simulink model "controller_tuning"  (R2020a)
settings: Solver=VariableStepAuto  StartTime=0.0  StopTime=10.0  RelTol=1e-3
model workspace (MAT data in the model file):
  DM0 = [1.094  0.6666; 0.3097  0.2601; -0.2633  0.1218; -0.351  0.6966; -0.105  0.4764; -0.3242  -0.09756; 0.796  1.029; 0.2022  0.05678]
  G = tf
  G.Variable_ = 'z^-1'
  G.InputName_ = ["TRIlong"; "TRIlat"; "TRImed"; "BIClong"; "BICshort"; "BRA"; "shoulder reserve"; "elbow reserve"]
  G.InputUnit_ = [""; ""; ""; ""; ""; ""; ""; ""]
  G.OutputName_ = ["y(1)"; "y(2)"]
  G.OutputUnit_ = [""; ""]
  G.Name_ = 'sys9'
  G.IOSize_ = [2 8]
  G.Data_ = ltipack.tfdata
  G.Data_.num{1,1} = [0 -0.00125852005922 -0.00123969277085 0.00578303193573 -0.00214602833438 -0.00815494705012 0.0108004774488 -0.0048408303984 0.000317114183203 0.000131024551851]
  G.Data_.num{2,1} = [0 -1.78877461201 3.42269225285 -0.172240731746 -4.80550166472 5.61225680994 -4.36357973513 4.54900861654 -3.65235478567 1.19849686118]
  G.Data_.num{1,2} = [0 0.0298263266299 -0.05603494088 0.00949204168653 0.0313146678964 0.0133073865004 -0.0557080006374 0.0253256021985 0.0130251372604 -0.00928844893676]
  G.Data_.num{2,2} = [0 6.78283210007 -16.0998067341 6.29571390083 14.1517930939 -18.338769316 15.0577755183 -18.5075343986 16.3599337451 -5.7019804007]
  G.Data_.num{1,3} = [0 -0.0274580753918 0.046649778889 0.000219075801083 -0.0277627580393 -0.0275977505479 0.0648552045639 -0.0245133704063 -0.0166522040766 0.0113266772791]
  G.Data_.num{2,3} = [0 -7.30509401763 17.0847598655 -6.42957231831 -15.715976147 21.2307859184 -18.337456702 20.0855611081 -15.011225285 4.39826116622]
  G.Data_.num{1,4} = [0 -0.000892023297362 0.00174771311212 -5.02626521608e-05 -0.0020036315742 0.000859099403795 0.00133312807044 -0.00136865103822 0.000340032171244 3.78324308943e-06]
  G.Data_.num{2,4} = [0 -0.125954978135 0.32847363204 -0.172297865784 -0.275766220436 0.382500727314 -0.353411491272 0.691035305427 -0.761724888908 0.287146907417]
  G.Data_.num{1,5} = [0 -0.00769047181105 0.0200271669402 -0.0171499217797 -0.0017607521966 0.0110210193173 -0.00610528432784 0.00273344797859 -0.00365422344999 0.00163564285109]
  G.Data_.num{2,5} = [0 -0.595361713331 0.656194025324 -0.708001157476 2.48746014578 -4.19785050587 4.1108803772 -2.57579141198 0.647172525737 0.175305987775]
  G.Data_.num{1,6} = [0 0.0106958101176 -0.0156960010931 -0.00894123836845 0.0450636393289 -0.0437527767735 0.00495298305972 0.0244991267401 -0.0226105055791 0.00832888442118]
  G.Data_.num{2,6} = [0 7.63813053731 -16.0040222918 8.78360619231 -0.807775906777 6.14010716966 -5.6743918868 -9.51802269738 16.2988522235 -6.85648806661]
  G.Data_.num{1,7} = [0 0.0096689266463 -0.0352403034351 0.0530644872076 -0.0277649986769 -0.0217759796863 0.0428504114816 -0.0292889462176 0.0114475784774 -0.00257741725747]
  G.Data_.num{2,7} = [0 0.705264065553 0.136559901801 -0.466566874265 -6.64333058905 16.0560931678 -19.450434008 16.8727296984 -9.81674981039 2.60643162571]
  G.Data_.num{1,8} = [0 -0.288241005177 0.902709439389 -0.75873047364 -0.65955283102 1.79703167037 -1.30558234166 0.128044890915 0.32409931535 -0.138466743751]
  G.Data_.num{2,8} = [0 -43.8066730621 155.493123951 -278.509814702 470.342011324 -720.208447619 693.978256442 -309.311208705 0.183476450966 31.8392957397]
  G.Data_.den{1,1} = [1 -3.44110275617 4.07951037305 -1.37498385443 -0.519157706389 -0.282617710591 0.517166185053 0.784556988423 -1.17222288306 0.408852682884]
  G.Data_.den{2,1} = [1 -3.44110275617 4.07951037305 -1.37498385443 -0.519157706389 -0.282617710591 0.517166185053 0.784556988423 -1.17222288306 0.408852682884]
  G.Data_.den{1,2} = [1 -3.44110275617 4.07951037305 -1.37498385443 -0.519157706389 -0.282617710591 0.517166185053 0.784556988423 -1.17222288306 0.408852682884]
  G.Data_.den{2,2} = [1 -3.44110275617 4.07951037305 -1.37498385443 -0.519157706389 -0.282617710591 0.517166185053 0.784556988423 -1.17222288306 0.408852682884]
  G.Data_.den{1,3} = [1 -3.44110275617 4.07951037305 -1.37498385443 -0.519157706389 -0.282617710591 0.517166185053 0.784556988423 -1.17222288306 0.408852682884]
  G.Data_.den{2,3} = [1 -3.44110275617 4.07951037305 -1.37498385443 -0.519157706389 -0.282617710591 0.517166185053 0.784556988423 -1.17222288306 0.408852682884]
  G.Data_.den{1,4} = [1 -3.44110275617 4.07951037305 -1.37498385443 -0.519157706389 -0.282617710591 0.517166185053 0.784556988423 -1.17222288306 0.408852682884]
  G.Data_.den{2,4} = [1 -3.44110275617 4.07951037305 -1.37498385443 -0.519157706389 -0.282617710591 0.517166185053 0.784556988423 -1.17222288306 0.408852682884]
  G.Data_.den{1,5} = [1 -3.44110275617 4.07951037305 -1.37498385443 -0.519157706389 -0.282617710591 0.517166185053 0.784556988423 -1.17222288306 0.408852682884]
  G.Data_.den{2,5} = [1 -3.44110275617 4.07951037305 -1.37498385443 -0.519157706389 -0.282617710591 0.517166185053 0.784556988423 -1.17222288306 0.408852682884]
  G.Data_.den{1,6} = [1 -3.44110275617 4.07951037305 -1.37498385443 -0.519157706389 -0.282617710591 0.517166185053 0.784556988423 -1.17222288306 0.408852682884]
  G.Data_.den{2,6} = [1 -3.44110275617 4.07951037305 -1.37498385443 -0.519157706389 -0.282617710591 0.517166185053 0.784556988423 -1.17222288306 0.408852682884]
  G.Data_.den{1,7} = [1 -3.44110275617 4.07951037305 -1.37498385443 -0.519157706389 -0.282617710591 0.517166185053 0.784556988423 -1.17222288306 0.408852682884]
  G.Data_.den{2,7} = [1 -3.44110275617 4.07951037305 -1.37498385443 -0.519157706389 -0.282617710591 0.517166185053 0.784556988423 -1.17222288306 0.408852682884]
  G.Data_.den{1,8} = [1 -3.44110275617 4.07951037305 -1.37498385443 -0.519157706389 -0.282617710591 0.517166185053 0.784556988423 -1.17222288306 0.408852682884]
  G.Data_.den{2,8} = [1 -3.44110275617 4.07951037305 -1.37498385443 -0.519157706389 -0.282617710591 0.517166185053 0.784556988423 -1.17222288306 0.408852682884]
  G.Data_.Delay.Input = [0; 0; 0; 0; 0; 0; 0; 0]
  G.Data_.Delay.Output = [0; 0]
  G.Data_.Delay.IO = [0  0  0  0  0  0  0  0; 0  0  0  0  0  0  0  0]
  G.Data_.Ts = 0.001
  Ts = 0.001
  controllers{1} = tunablePID
  controllers{1}.Kp_ = param.Continuous
  controllers{1}.Kp_.Size_ = [1 1]
  controllers{1}.Kp_.Value_ = 0
  controllers{1}.Kp_.pID = paramid.Variable
  controllers{1}.Kp_.pID.Name = 'Kp'
  controllers{1}.Ki_ = param.Continuous
  controllers{1}.Ki_.Size_ = [1 1]
  controllers{1}.Ki_.Value_ = 0.001
  controllers{1}.Ki_.pID = paramid.Variable
  controllers{1}.Ki_.pID.Name = 'Ki'
  controllers{1}.Kd_ = param.Continuous
  controllers{1}.Kd_.Free_ = 0
  controllers{1}.Kd_.Size_ = [1 1]
  controllers{1}.Kd_.Value_ = 0
  controllers{1}.Kd_.pID = paramid.Variable
  controllers{1}.Kd_.pID.Name = 'Kd'
  controllers{1}.Tf_ = param.Continuous
  controllers{1}.Tf_.Minimum_ = 0
  controllers{1}.Tf_.Free_ = 0
  controllers{1}.Tf_.Size_ = [1 1]
  controllers{1}.Tf_.Value_ = 1
  controllers{1}.Tf_.pID = paramid.Variable
  controllers{1}.Tf_.pID.Name = 'Tf'
  controllers{1}.Name_ = 'PI1'
  controllers{1}.IOSize_ = [1 1]
  controllers{1}.Ts_ = 0.001
  controllers{1}.InputName_ = "p(1)"
  controllers{1}.OutputName_ = "TRIlong"
  controllers{2} = tunablePID
  controllers{2}.Kp_ = param.Continuous
  controllers{2}.Kp_.Size_ = [1 1]
  controllers{2}.Kp_.Value_ = 0
  controllers{2}.Kp_.pID = paramid.Variable
  controllers{2}.Kp_.pID.Name = 'Kp'
  controllers{2}.Ki_ = param.Continuous
  controllers{2}.Ki_.Size_ = [1 1]
  controllers{2}.Ki_.Value_ = 0.001
  controllers{2}.Ki_.pID = paramid.Variable
  controllers{2}.Ki_.pID.Name = 'Ki'
  controllers{2}.Kd_ = param.Continuous
  controllers{2}.Kd_.Free_ = 0
  controllers{2}.Kd_.Size_ = [1 1]
  controllers{2}.Kd_.Value_ = 0
  controllers{2}.Kd_.pID = paramid.Variable
  controllers{2}.Kd_.pID.Name = 'Kd'
  controllers{2}.Tf_ = param.Continuous
  controllers{2}.Tf_.Minimum_ = 0
  controllers{2}.Tf_.Free_ = 0
  controllers{2}.Tf_.Size_ = [1 1]
  controllers{2}.Tf_.Value_ = 1
  controllers{2}.Tf_.pID = paramid.Variable
  controllers{2}.Tf_.pID.Name = 'Tf'
  controllers{2}.Name_ = 'PI2'
  controllers{2}.IOSize_ = [1 1]
  controllers{2}.Ts_ = 0.001
  controllers{2}.InputName_ = "p(2)"
  controllers{2}.OutputName_ = "TRIlat"
  controllers{3} = tunablePID
  controllers{3}.Kp_ = param.Continuous
  controllers{3}.Kp_.Size_ = [1 1]
  controllers{3}.Kp_.Value_ = 0
  controllers{3}.Kp_.pID = paramid.Variable
  controllers{3}.Kp_.pID.Name = 'Kp'
  controllers{3}.Ki_ = param.Continuous
  controllers{3}.Ki_.Size_ = [1 1]
  controllers{3}.Ki_.Value_ = 0.001
  controllers{3}.Ki_.pID = paramid.Variable
  controllers{3}.Ki_.pID.Name = 'Ki'
  controllers{3}.Kd_ = param.Continuous
  controllers{3}.Kd_.Free_ = 0
  controllers{3}.Kd_.Size_ = [1 1]
  controllers{3}.Kd_.Value_ = 0
  controllers{3}.Kd_.pID = paramid.Variable
  controllers{3}.Kd_.pID.Name = 'Kd'
  controllers{3}.Tf_ = param.Continuous
  controllers{3}.Tf_.Minimum_ = 0
  controllers{3}.Tf_.Free_ = 0
  controllers{3}.Tf_.Size_ = [1 1]
  controllers{3}.Tf_.Value_ = 1
  controllers{3}.Tf_.pID = paramid.Variable
  controllers{3}.Tf_.pID.Name = 'Tf'
  controllers{3}.Name_ = 'PI3'
  controllers{3}.IOSize_ = [1 1]
  controllers{3}.Ts_ = 0.001
  controllers{3}.InputName_ = "p(3)"
  controllers{3}.OutputName_ = "TRImed"
  controllers{4} = tunablePID
  controllers{4}.Kp_ = param.Continuous
  controllers{4}.Kp_.Size_ = [1 1]
  controllers{4}.Kp_.Value_ = 0
  controllers{4}.Kp_.pID = paramid.Variable
  controllers{4}.Kp_.pID.Name = 'Kp'
  controllers{4}.Ki_ = param.Continuous
  controllers{4}.Ki_.Size_ = [1 1]
  controllers{4}.Ki_.Value_ = 0.001
  controllers{4}.Ki_.pID = paramid.Variable
  controllers{4}.Ki_.pID.Name = 'Ki'
  controllers{4}.Kd_ = param.Continuous
  controllers{4}.Kd_.Free_ = 0
  controllers{4}.Kd_.Size_ = [1 1]
  controllers{4}.Kd_.Value_ = 0
  controllers{4}.Kd_.pID = paramid.Variable
  controllers{4}.Kd_.pID.Name = 'Kd'
  controllers{4}.Tf_ = param.Continuous
  controllers{4}.Tf_.Minimum_ = 0
  controllers{4}.Tf_.Free_ = 0
  controllers{4}.Tf_.Size_ = [1 1]
  controllers{4}.Tf_.Value_ = 1
  controllers{4}.Tf_.pID = paramid.Variable
  controllers{4}.Tf_.pID.Name = 'Tf'
  controllers{4}.Name_ = 'PI4'
  controllers{4}.IOSize_ = [1 1]
  controllers{4}.Ts_ = 0.001
  controllers{4}.InputName_ = "p(4)"
  controllers{4}.OutputName_ = "BIClong"
  controllers{5} = tunablePID
  controllers{5}.Kp_ = param.Continuous
  controllers{5}.Kp_.Size_ = [1 1]
  controllers{5}.Kp_.Value_ = 0
  controllers{5}.Kp_.pID = paramid.Variable
  controllers{5}.Kp_.pID.Name = 'Kp'
  controllers{5}.Ki_ = param.Continuous
  controllers{5}.Ki_.Size_ = [1 1]
  controllers{5}.Ki_.Value_ = 0.001
  controllers{5}.Ki_.pID = paramid.Variable
  controllers{5}.Ki_.pID.Name = 'Ki'
  controllers{5}.Kd_ = param.Continuous
  controllers{5}.Kd_.Free_ = 0
  controllers{5}.Kd_.Size_ = [1 1]
  controllers{5}.Kd_.Value_ = 0
  controllers{5}.Kd_.pID = paramid.Variable
  controllers{5}.Kd_.pID.Name = 'Kd'
  controllers{5}.Tf_ = param.Continuous
  controllers{5}.Tf_.Minimum_ = 0
  controllers{5}.Tf_.Free_ = 0
  controllers{5}.Tf_.Size_ = [1 1]
  controllers{5}.Tf_.Value_ = 1
  controllers{5}.Tf_.pID = paramid.Variable
  controllers{5}.Tf_.pID.Name = 'Tf'
  controllers{5}.Name_ = 'PI5'
  controllers{5}.IOSize_ = [1 1]
  controllers{5}.Ts_ = 0.001
  controllers{5}.InputName_ = "p(5)"
  controllers{5}.OutputName_ = "BICshort"
  controllers{6} = tunablePID
  controllers{6}.Kp_ = param.Continuous
  controllers{6}.Kp_.Size_ = [1 1]
  controllers{6}.Kp_.Value_ = 0
  controllers{6}.Kp_.pID = paramid.Variable
  controllers{6}.Kp_.pID.Name = 'Kp'
  controllers{6}.Ki_ = param.Continuous
  controllers{6}.Ki_.Size_ = [1 1]
  controllers{6}.Ki_.Value_ = 0.001
  controllers{6}.Ki_.pID = paramid.Variable
  controllers{6}.Ki_.pID.Name = 'Ki'
  controllers{6}.Kd_ = param.Continuous
  controllers{6}.Kd_.Free_ = 0
  controllers{6}.Kd_.Size_ = [1 1]
  controllers{6}.Kd_.Value_ = 0
  controllers{6}.Kd_.pID = paramid.Variable
  controllers{6}.Kd_.pID.Name = 'Kd'
  controllers{6}.Tf_ = param.Continuous
  controllers{6}.Tf_.Minimum_ = 0
  controllers{6}.Tf_.Free_ = 0
  controllers{6}.Tf_.Size_ = [1 1]
  controllers{6}.Tf_.Value_ = 1
  controllers{6}.Tf_.pID = paramid.Variable
  controllers{6}.Tf_.pID.Name = 'Tf'
  controllers{6}.Name_ = 'PI6'
  controllers{6}.IOSize_ = [1 1]
  controllers{6}.Ts_ = 0.001
  controllers{6}.InputName_ = "p(6)"
  controllers{6}.OutputName_ = "BRA"
  controllers{7} = tunablePID
  controllers{7}.Kp_ = param.Continuous
  controllers{7}.Kp_.Size_ = [1 1]
  controllers{7}.Kp_.Value_ = 0
  controllers{7}.Kp_.pID = paramid.Variable
  controllers{7}.Kp_.pID.Name = 'Kp'
  controllers{7}.Ki_ = param.Continuous
  controllers{7}.Ki_.Size_ = [1 1]
  controllers{7}.Ki_.Value_ = 0.001
  controllers{7}.Ki_.pID = paramid.Variable
  controllers{7}.Ki_.pID.Name = 'Ki'
  controllers{7}.Kd_ = param.Continuous
  controllers{7}.Kd_.Free_ = 0
  controllers{7}.Kd_.Size_ = [1 1]
  controllers{7}.Kd_.Value_ = 0
  controllers{7}.Kd_.pID = paramid.Variable
  controllers{7}.Kd_.pID.Name = 'Kd'
  controllers{7}.Tf_ = param.Continuous
  controllers{7}.Tf_.Minimum_ = 0
  controllers{7}.Tf_.Free_ = 0
  controllers{7}.Tf_.Size_ = [1 1]
  controllers{7}.Tf_.Value_ = 1
  controllers{7}.Tf_.pID = paramid.Variable
  controllers{7}.Tf_.pID.Name = 'Tf'
  controllers{7}.Name_ = 'PI7'
  controllers{7}.IOSize_ = [1 1]
  controllers{7}.Ts_ = 0.001
  controllers{7}.InputName_ = "p(7)"
  controllers{7}.OutputName_ = "shoulder reserve"
  controllers{8} = tunablePID
  controllers{8}.Kp_ = param.Continuous
  controllers{8}.Kp_.Size_ = [1 1]
  controllers{8}.Kp_.Value_ = 0
  controllers{8}.Kp_.pID = paramid.Variable
  controllers{8}.Kp_.pID.Name = 'Kp'
  controllers{8}.Ki_ = param.Continuous
  controllers{8}.Ki_.Size_ = [1 1]
  controllers{8}.Ki_.Value_ = 0.001
  controllers{8}.Ki_.pID = paramid.Variable
  controllers{8}.Ki_.pID.Name = 'Ki'
  controllers{8}.Kd_ = param.Continuous
  controllers{8}.Kd_.Free_ = 0
  controllers{8}.Kd_.Size_ = [1 1]
  controllers{8}.Kd_.Value_ = 0
  controllers{8}.Kd_.pID = paramid.Variable
  controllers{8}.Kd_.pID.Name = 'Kd'
  controllers{8}.Tf_ = param.Continuous
  controllers{8}.Tf_.Minimum_ = 0
  controllers{8}.Tf_.Free_ = 0
  controllers{8}.Tf_.Size_ = [1 1]
  controllers{8}.Tf_.Value_ = 1
  controllers{8}.Tf_.pID = paramid.Variable
  controllers{8}.Tf_.pID.Name = 'Tf'
  controllers{8}.Name_ = 'PI8'
  controllers{8}.IOSize_ = [1 1]
  controllers{8}.Ts_ = 0.001
  controllers{8}.InputName_ = "p(8)"
  controllers{8}.OutputName_ = "elbow reserve"
values from neighbouring files (symbols this model uses):
  D = tunableGain('Decoupler', numinputs, numoutputs)    [closed_loop_controller_tuning.m]    (also in steptester.m)
  G = sys_tf    [closed_loop_controller_tuning.m]    (also in steptester.m)
undefined symbols (not defined in the file or in its folder): Tdio
libraries: cstextras x20, simulink x16, simulink_extras x2
settings Model: Creator=Jaxton  LastModifiedBy=Jaxton

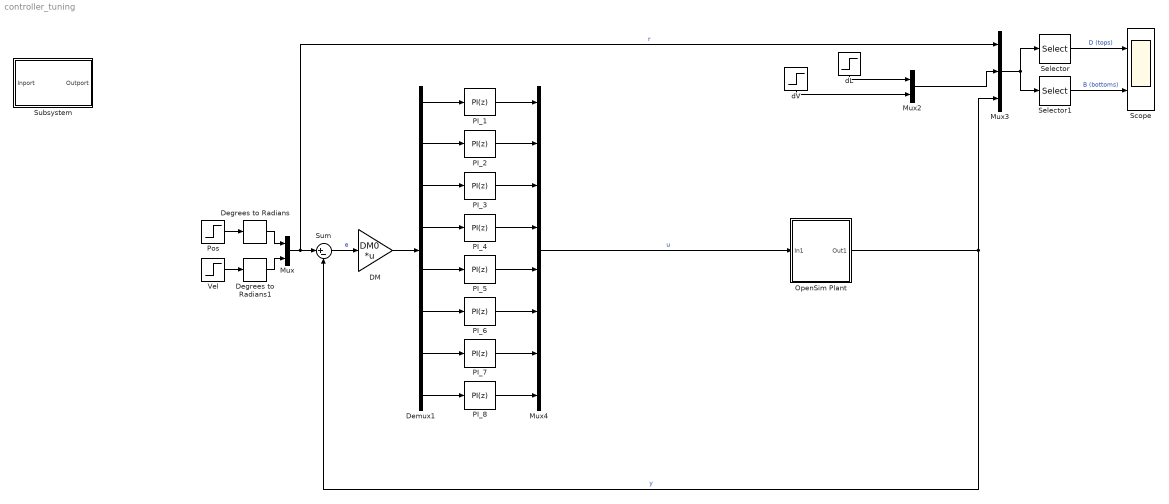
== system controller_tuning ==
  DM : Gain  Gain=DM0  Multiplication=Matrix(K*u)
  Degrees to Radians : simulink_extras/Transformations/Degrees to Radians
  Degrees to Radians1 : simulink_extras/Transformations/Degrees to Radians
  Demux1 : Demux  Outputs=8
  Mux : Mux  Inputs=2
  Mux2 : Mux  Inputs=2
  Mux3 : Mux  Inputs=3
  Mux4 : Mux  Inputs=8
  OpenSim Plant : Subsystem  BlockChoice=CSS  mask(LTI Block){sys=G, IC=[]}
      mask prompts: sys "Control:simulink:LTIMaskLabel1"; IC "Control:simulink:LTIMaskLabel2"
      mask help: Control:simulink:LTIMaskDescription
      mask init:
      | try
      |    % read data to initialize mask variables
      |    [D,Ts,Tdi,Tdo,Tdio,x0,sysname]=...
      |       ltimask('Initialize',gcb,sys,IC);
      |    % update contents
      |    model = bdroot;
      |    df = get_param(model,'dirty');
      |    ltimask('UpdateDiagram',gcb,D,Ts,Tdio);
      |    try      
      |       % Attempt to modify locked library -> error
      |       % Makes block show ??? when loading CSTBLOCKS
      |       % for the first time
      |       set_param(model,'dirty',df)
      |    end
      | catch ME
      |    sys = [];  IC = [];   sysname = '???';
      |    throw(ME)
      | end
      mask Help: eval('ctrlguihelp(''ltisystemblock'');')
      mask Callback sys: ltimask('MaskLTICallback',gcb);
      mask Display: disp(sysname)
  PI_1 : simulink/Continuous/PID Controller  Controller=PI  Form=Parallel  TimeDomain=Discrete-time  UseExternalTs=off  SampleTime=-1  IntegratorMethod=Forward Euler  FilterMethod=Forward Euler  ControllerParametersSource=internal  P=-0.385  I=-0.958  D=0  UseFilter=on  N=100  TunerSelectOption=Transfer Function Based (PID Tuner App)  InitialConditionSource=internal  InitialConditionForIntegrator=0  InitialConditionForFilter=0  DifferentiatorICPrevScaledInput=0  ExternalReset=none  TrackingMode=off  Kt=1  LimitOutput=off  UpperSaturationLimit=inf  LowerSaturationLimit=-inf  LinearizeAsGain=off  AntiWindupMode=none  Kb=1  POutMin=[]  POutMax=[]  IOutMin=[]  IOutMax=[]  DOutMin=[]  DOutMax=[]  NOutMin=[]  NOutMax=[]  SumOutMin=[]  SumOutMax=[]  SaturationOutMin=[]  SaturationOutMax=[]  PParamMin=[]  PParamMax=[]  IParamMin=[]  IParamMax=[]  DParamMin=[]  DParamMax=[]  NParamMin=[]  NParamMax=[]  KbParamMin=[]  KbParamMax=[]  KtParamMin=[]  KtParamMax=[]  KbOutMin=[]  KbOutMax=[]  KtOutMin=[]  KtOutMax=[]  IntegratorOutMin=[]  IntegratorOutMax=[]  FilterOutMin=[]  FilterOutMax=[]  SumI1OutMin=[]  SumI1OutMax=[]  SumI2OutMin=[]  SumI2OutMax=[]  SumI3OutMin=[]  SumI3OutMax=[]  SumI4OutMin=[]  SumI4OutMax=[]  SumDOutMin=[]  SumDOutMax=[]  DifferentiatorOutMin=[]  DifferentiatorOutMax=[]  FilterDiffOutCoefMin=[]  FilterDiffOutCoefMax=[]  ReciprocalOutMin=[]  ReciprocalOutMax=[]  SumDenOutMin=[]  SumDenOutMax=[]  SumNumOutMin=[]  SumNumOutMax=[]  DivideOutMin=[]  DivideOutMax=[]  UdiffTsProdOutMin=[]  UdiffTsProdOutMax=[]  NTsProdOutMin=[]  NTsProdOutMax=[]  UintegralTsProdOutMin=[]  UintegralTsProdOutMax=[]  UngainTsProdOutMin=[]  UngainTsProdOutMax=[]  IntegratorContinuousStateAttributes=''  IntegratorStateMustResolveToSignalObject=off  IntegratorRTWStateStorageClass=Auto  FilterContinuousStateAttributes=''  FilterStateMustResolveToSignalObject=off  FilterRTWStateStorageClass=Auto  ParallelPVariant=InternalParameters  IdealPVariant=Disabled  IVariant=InternalParameters  DVariant=Disabled  IntegratorVariant=Discrete  SatVariant=Disabled  AWVariant=Passthrough  PCopyVariant=Disabled  TRVariant=Disabled  FdbkBlocksVariant=Forward  IdealPFdbkVariant=Disabled  SatFdbkVariant=Disabled  DerivativeFilterVariant=Disabled  NVariant=Disabled  NCopyVariant=Disabled_SignalSpec  FilterICVariant=Disabled  IntegratorICVariant=InternalICs  ExternalResetVariant=Disabled  TRSumVariant=Passthrough  SumFdbkVariant=Disabled  SumVariant=Sum_PI  TsampFilterVariant=InternalTs  TsampNgainVariant=Passthrough  TsampIntegralVariant=Passthrough
  PI_2 : simulink/Continuous/PID Controller  Controller=PI  Form=Parallel  TimeDomain=Discrete-time  UseExternalTs=off  SampleTime=-1  IntegratorMethod=Forward Euler  FilterMethod=Forward Euler  ControllerParametersSource=internal  P=0.0215  I=-0.0795  D=0  UseFilter=on  N=100  TunerSelectOption=Transfer Function Based (PID Tuner App)  InitialConditionSource=internal  InitialConditionForIntegrator=0  InitialConditionForFilter=0  DifferentiatorICPrevScaledInput=0  ExternalReset=none  TrackingMode=off  Kt=1  LimitOutput=off  UpperSaturationLimit=inf  LowerSaturationLimit=-inf  LinearizeAsGain=off  AntiWindupMode=none  Kb=1  POutMin=[]  POutMax=[]  IOutMin=[]  IOutMax=[]  DOutMin=[]  DOutMax=[]  NOutMin=[]  NOutMax=[]  SumOutMin=[]  SumOutMax=[]  SaturationOutMin=[]  SaturationOutMax=[]  PParamMin=[]  PParamMax=[]  IParamMin=[]  IParamMax=[]  DParamMin=[]  DParamMax=[]  NParamMin=[]  NParamMax=[]  KbParamMin=[]  KbParamMax=[]  KtParamMin=[]  KtParamMax=[]  KbOutMin=[]  KbOutMax=[]  KtOutMin=[]  KtOutMax=[]  IntegratorOutMin=[]  IntegratorOutMax=[]  FilterOutMin=[]  FilterOutMax=[]  SumI1OutMin=[]  SumI1OutMax=[]  SumI2OutMin=[]  SumI2OutMax=[]  SumI3OutMin=[]  SumI3OutMax=[]  SumI4OutMin=[]  SumI4OutMax=[]  SumDOutMin=[]  SumDOutMax=[]  DifferentiatorOutMin=[]  DifferentiatorOutMax=[]  FilterDiffOutCoefMin=[]  FilterDiffOutCoefMax=[]  ReciprocalOutMin=[]  ReciprocalOutMax=[]  SumDenOutMin=[]  SumDenOutMax=[]  SumNumOutMin=[]  SumNumOutMax=[]  DivideOutMin=[]  DivideOutMax=[]  UdiffTsProdOutMin=[]  UdiffTsProdOutMax=[]  NTsProdOutMin=[]  NTsProdOutMax=[]  UintegralTsProdOutMin=[]  UintegralTsProdOutMax=[]  UngainTsProdOutMin=[]  UngainTsProdOutMax=[]  IntegratorContinuousStateAttributes=''  IntegratorStateMustResolveToSignalObject=off  IntegratorRTWStateStorageClass=Auto  FilterContinuousStateAttributes=''  FilterStateMustResolveToSignalObject=off  FilterRTWStateStorageClass=Auto  ParallelPVariant=InternalParameters  IdealPVariant=Disabled  IVariant=InternalParameters  DVariant=Disabled  IntegratorVariant=Discrete  SatVariant=Disabled  AWVariant=Passthrough  PCopyVariant=Disabled  TRVariant=Disabled  FdbkBlocksVariant=Forward  IdealPFdbkVariant=Disabled  SatFdbkVariant=Disabled  DerivativeFilterVariant=Disabled  NVariant=Disabled  NCopyVariant=Disabled_SignalSpec  FilterICVariant=Disabled  IntegratorICVariant=InternalICs  ExternalResetVariant=Disabled  TRSumVariant=Passthrough  SumFdbkVariant=Disabled  SumVariant=Sum_PI  TsampFilterVariant=InternalTs  TsampNgainVariant=Passthrough  TsampIntegralVariant=Passthrough
  PI_3 : simulink/Continuous/PID Controller  Controller=PI  Form=Parallel  TimeDomain=Discrete-time  UseExternalTs=off  SampleTime=-1  IntegratorMethod=Forward Euler  FilterMethod=Forward Euler  ControllerParametersSource=internal  P=0.117  I=0.232  D=0  UseFilter=on  N=100  TunerSelectOption=Transfer Function Based (PID Tuner App)  InitialConditionSource=internal  InitialConditionForIntegrator=0  InitialConditionForFilter=0  DifferentiatorICPrevScaledInput=0  ExternalReset=none  TrackingMode=off  Kt=1  LimitOutput=off  UpperSaturationLimit=inf  LowerSaturationLimit=-inf  LinearizeAsGain=off  AntiWindupMode=none  Kb=1  POutMin=[]  POutMax=[]  IOutMin=[]  IOutMax=[]  DOutMin=[]  DOutMax=[]  NOutMin=[]  NOutMax=[]  SumOutMin=[]  SumOutMax=[]  SaturationOutMin=[]  SaturationOutMax=[]  PParamMin=[]  PParamMax=[]  IParamMin=[]  IParamMax=[]  DParamMin=[]  DParamMax=[]  NParamMin=[]  NParamMax=[]  KbParamMin=[]  KbParamMax=[]  KtParamMin=[]  KtParamMax=[]  KbOutMin=[]  KbOutMax=[]  KtOutMin=[]  KtOutMax=[]  IntegratorOutMin=[]  IntegratorOutMax=[]  FilterOutMin=[]  FilterOutMax=[]  SumI1OutMin=[]  SumI1OutMax=[]  SumI2OutMin=[]  SumI2OutMax=[]  SumI3OutMin=[]  SumI3OutMax=[]  SumI4OutMin=[]  SumI4OutMax=[]  SumDOutMin=[]  SumDOutMax=[]  DifferentiatorOutMin=[]  DifferentiatorOutMax=[]  FilterDiffOutCoefMin=[]  FilterDiffOutCoefMax=[]  ReciprocalOutMin=[]  ReciprocalOutMax=[]  SumDenOutMin=[]  SumDenOutMax=[]  SumNumOutMin=[]  SumNumOutMax=[]  DivideOutMin=[]  DivideOutMax=[]  UdiffTsProdOutMin=[]  UdiffTsProdOutMax=[]  NTsProdOutMin=[]  NTsProdOutMax=[]  UintegralTsProdOutMin=[]  UintegralTsProdOutMax=[]  UngainTsProdOutMin=[]  UngainTsProdOutMax=[]  IntegratorContinuousStateAttributes=''  IntegratorStateMustResolveToSignalObject=off  IntegratorRTWStateStorageClass=Auto  FilterContinuousStateAttributes=''  FilterStateMustResolveToSignalObject=off  FilterRTWStateStorageClass=Auto  ParallelPVariant=InternalParameters  IdealPVariant=Disabled  IVariant=InternalParameters  DVariant=Disabled  IntegratorVariant=Discrete  SatVariant=Disabled  AWVariant=Passthrough  PCopyVariant=Disabled  TRVariant=Disabled  FdbkBlocksVariant=Forward  IdealPFdbkVariant=Disabled  SatFdbkVariant=Disabled  DerivativeFilterVariant=Disabled  NVariant=Disabled  NCopyVariant=Disabled_SignalSpec  FilterICVariant=Disabled  IntegratorICVariant=InternalICs  ExternalResetVariant=Disabled  TRSumVariant=Passthrough  SumFdbkVariant=Disabled  SumVariant=Sum_PI  TsampFilterVariant=InternalTs  TsampNgainVariant=Passthrough  TsampIntegralVariant=Passthrough
  PI_4 : simulink/Continuous/PID Controller  Controller=PI  Form=Parallel  TimeDomain=Discrete-time  UseExternalTs=off  SampleTime=-1  IntegratorMethod=Forward Euler  FilterMethod=Forward Euler  ControllerParametersSource=internal  P=-1.99  I=-2.96  D=0  UseFilter=on  N=100  TunerSelectOption=Transfer Function Based (PID Tuner App)  InitialConditionSource=internal  InitialConditionForIntegrator=0  InitialConditionForFilter=0  DifferentiatorICPrevScaledInput=0  ExternalReset=none  TrackingMode=off  Kt=1  LimitOutput=off  UpperSaturationLimit=inf  LowerSaturationLimit=-inf  LinearizeAsGain=off  AntiWindupMode=none  Kb=1  POutMin=[]  POutMax=[]  IOutMin=[]  IOutMax=[]  DOutMin=[]  DOutMax=[]  NOutMin=[]  NOutMax=[]  SumOutMin=[]  SumOutMax=[]  SaturationOutMin=[]  SaturationOutMax=[]  PParamMin=[]  PParamMax=[]  IParamMin=[]  IParamMax=[]  DParamMin=[]  DParamMax=[]  NParamMin=[]  NParamMax=[]  KbParamMin=[]  KbParamMax=[]  KtParamMin=[]  KtParamMax=[]  KbOutMin=[]  KbOutMax=[]  KtOutMin=[]  KtOutMax=[]  IntegratorOutMin=[]  IntegratorOutMax=[]  FilterOutMin=[]  FilterOutMax=[]  SumI1OutMin=[]  SumI1OutMax=[]  SumI2OutMin=[]  SumI2OutMax=[]  SumI3OutMin=[]  SumI3OutMax=[]  SumI4OutMin=[]  SumI4OutMax=[]  SumDOutMin=[]  SumDOutMax=[]  DifferentiatorOutMin=[]  DifferentiatorOutMax=[]  FilterDiffOutCoefMin=[]  FilterDiffOutCoefMax=[]  ReciprocalOutMin=[]  ReciprocalOutMax=[]  SumDenOutMin=[]  SumDenOutMax=[]  SumNumOutMin=[]  SumNumOutMax=[]  DivideOutMin=[]  DivideOutMax=[]  UdiffTsProdOutMin=[]  UdiffTsProdOutMax=[]  NTsProdOutMin=[]  NTsProdOutMax=[]  UintegralTsProdOutMin=[]  UintegralTsProdOutMax=[]  UngainTsProdOutMin=[]  UngainTsProdOutMax=[]  IntegratorContinuousStateAttributes=''  IntegratorStateMustResolveToSignalObject=off  IntegratorRTWStateStorageClass=Auto  FilterContinuousStateAttributes=''  FilterStateMustResolveToSignalObject=off  FilterRTWStateStorageClass=Auto  ParallelPVariant=InternalParameters  IdealPVariant=Disabled  IVariant=InternalParameters  DVariant=Disabled  IntegratorVariant=Discrete  SatVariant=Disabled  AWVariant=Passthrough  PCopyVariant=Disabled  TRVariant=Disabled  FdbkBlocksVariant=Forward  IdealPFdbkVariant=Disabled  SatFdbkVariant=Disabled  DerivativeFilterVariant=Disabled  NVariant=Disabled  NCopyVariant=Disabled_SignalSpec  FilterICVariant=Disabled  IntegratorICVariant=InternalICs  ExternalResetVariant=Disabled  TRSumVariant=Passthrough  SumFdbkVariant=Disabled  SumVariant=Sum_PI  TsampFilterVariant=InternalTs  TsampNgainVariant=Passthrough  TsampIntegralVariant=Passthrough
  PI_5 : simulink/Continuous/PID Controller  Controller=PI  Form=Parallel  TimeDomain=Discrete-time  UseExternalTs=off  SampleTime=-1  IntegratorMethod=Forward Euler  FilterMethod=Forward Euler  ControllerParametersSource=internal  P=0.286  I=-0.516  D=0  UseFilter=on  N=100  TunerSelectOption=Transfer Function Based (PID Tuner App)  InitialConditionSource=internal  InitialConditionForIntegrator=0  InitialConditionForFilter=0  DifferentiatorICPrevScaledInput=0  ExternalReset=none  TrackingMode=off  Kt=1  LimitOutput=off  UpperSaturationLimit=inf  LowerSaturationLimit=-inf  LinearizeAsGain=off  AntiWindupMode=none  Kb=1  POutMin=[]  POutMax=[]  IOutMin=[]  IOutMax=[]  DOutMin=[]  DOutMax=[]  NOutMin=[]  NOutMax=[]  SumOutMin=[]  SumOutMax=[]  SaturationOutMin=[]  SaturationOutMax=[]  PParamMin=[]  PParamMax=[]  IParamMin=[]  IParamMax=[]  DParamMin=[]  DParamMax=[]  NParamMin=[]  NParamMax=[]  KbParamMin=[]  KbParamMax=[]  KtParamMin=[]  KtParamMax=[]  KbOutMin=[]  KbOutMax=[]  KtOutMin=[]  KtOutMax=[]  IntegratorOutMin=[]  IntegratorOutMax=[]  FilterOutMin=[]  FilterOutMax=[]  SumI1OutMin=[]  SumI1OutMax=[]  SumI2OutMin=[]  SumI2OutMax=[]  SumI3OutMin=[]  SumI3OutMax=[]  SumI4OutMin=[]  SumI4OutMax=[]  SumDOutMin=[]  SumDOutMax=[]  DifferentiatorOutMin=[]  DifferentiatorOutMax=[]  FilterDiffOutCoefMin=[]  FilterDiffOutCoefMax=[]  ReciprocalOutMin=[]  ReciprocalOutMax=[]  SumDenOutMin=[]  SumDenOutMax=[]  SumNumOutMin=[]  SumNumOutMax=[]  DivideOutMin=[]  DivideOutMax=[]  UdiffTsProdOutMin=[]  UdiffTsProdOutMax=[]  NTsProdOutMin=[]  NTsProdOutMax=[]  UintegralTsProdOutMin=[]  UintegralTsProdOutMax=[]  UngainTsProdOutMin=[]  UngainTsProdOutMax=[]  IntegratorContinuousStateAttributes=''  IntegratorStateMustResolveToSignalObject=off  IntegratorRTWStateStorageClass=Auto  FilterContinuousStateAttributes=''  FilterStateMustResolveToSignalObject=off  FilterRTWStateStorageClass=Auto  ParallelPVariant=InternalParameters  IdealPVariant=Disabled  IVariant=InternalParameters  DVariant=Disabled  IntegratorVariant=Discrete  SatVariant=Disabled  AWVariant=Passthrough  PCopyVariant=Disabled  TRVariant=Disabled  FdbkBlocksVariant=Forward  IdealPFdbkVariant=Disabled  SatFdbkVariant=Disabled  DerivativeFilterVariant=Disabled  NVariant=Disabled  NCopyVariant=Disabled_SignalSpec  FilterICVariant=Disabled  IntegratorICVariant=InternalICs  ExternalResetVariant=Disabled  TRSumVariant=Passthrough  SumFdbkVariant=Disabled  SumVariant=Sum_PI  TsampFilterVariant=InternalTs  TsampNgainVariant=Passthrough  TsampIntegralVariant=Passthrough
  PI_6 : simulink/Continuous/PID Controller  Controller=PI  Form=Parallel  TimeDomain=Discrete-time  UseExternalTs=off  SampleTime=-1  IntegratorMethod=Forward Euler  FilterMethod=Forward Euler  ControllerParametersSource=internal  P=-0.0726  I=-0.206  D=0  UseFilter=on  N=100  TunerSelectOption=Transfer Function Based (PID Tuner App)  InitialConditionSource=internal  InitialConditionForIntegrator=0  InitialConditionForFilter=0  DifferentiatorICPrevScaledInput=0  ExternalReset=none  TrackingMode=off  Kt=1  LimitOutput=off  UpperSaturationLimit=inf  LowerSaturationLimit=-inf  LinearizeAsGain=off  AntiWindupMode=none  Kb=1  POutMin=[]  POutMax=[]  IOutMin=[]  IOutMax=[]  DOutMin=[]  DOutMax=[]  NOutMin=[]  NOutMax=[]  SumOutMin=[]  SumOutMax=[]  SaturationOutMin=[]  SaturationOutMax=[]  PParamMin=[]  PParamMax=[]  IParamMin=[]  IParamMax=[]  DParamMin=[]  DParamMax=[]  NParamMin=[]  NParamMax=[]  KbParamMin=[]  KbParamMax=[]  KtParamMin=[]  KtParamMax=[]  KbOutMin=[]  KbOutMax=[]  KtOutMin=[]  KtOutMax=[]  IntegratorOutMin=[]  IntegratorOutMax=[]  FilterOutMin=[]  FilterOutMax=[]  SumI1OutMin=[]  SumI1OutMax=[]  SumI2OutMin=[]  SumI2OutMax=[]  SumI3OutMin=[]  SumI3OutMax=[]  SumI4OutMin=[]  SumI4OutMax=[]  SumDOutMin=[]  SumDOutMax=[]  DifferentiatorOutMin=[]  DifferentiatorOutMax=[]  FilterDiffOutCoefMin=[]  FilterDiffOutCoefMax=[]  ReciprocalOutMin=[]  ReciprocalOutMax=[]  SumDenOutMin=[]  SumDenOutMax=[]  SumNumOutMin=[]  SumNumOutMax=[]  DivideOutMin=[]  DivideOutMax=[]  UdiffTsProdOutMin=[]  UdiffTsProdOutMax=[]  NTsProdOutMin=[]  NTsProdOutMax=[]  UintegralTsProdOutMin=[]  UintegralTsProdOutMax=[]  UngainTsProdOutMin=[]  UngainTsProdOutMax=[]  IntegratorContinuousStateAttributes=''  IntegratorStateMustResolveToSignalObject=off  IntegratorRTWStateStorageClass=Auto  FilterContinuousStateAttributes=''  FilterStateMustResolveToSignalObject=off  FilterRTWStateStorageClass=Auto  ParallelPVariant=InternalParameters  IdealPVariant=Disabled  IVariant=InternalParameters  DVariant=Disabled  IntegratorVariant=Discrete  SatVariant=Disabled  AWVariant=Passthrough  PCopyVariant=Disabled  TRVariant=Disabled  FdbkBlocksVariant=Forward  IdealPFdbkVariant=Disabled  SatFdbkVariant=Disabled  DerivativeFilterVariant=Disabled  NVariant=Disabled  NCopyVariant=Disabled_SignalSpec  FilterICVariant=Disabled  IntegratorICVariant=InternalICs  ExternalResetVariant=Disabled  TRSumVariant=Passthrough  SumFdbkVariant=Disabled  SumVariant=Sum_PI  TsampFilterVariant=InternalTs  TsampNgainVariant=Passthrough  TsampIntegralVariant=Passthrough
  PI_7 : simulink/Continuous/PID Controller  Controller=PI  Form=Parallel  TimeDomain=Discrete-time  UseExternalTs=off  SampleTime=-1  IntegratorMethod=Forward Euler  FilterMethod=Forward Euler  ControllerParametersSource=internal  P=0.112  I=-1.79  D=0  UseFilter=on  N=100  TunerSelectOption=Transfer Function Based (PID Tuner App)  InitialConditionSource=internal  InitialConditionForIntegrator=0  InitialConditionForFilter=0  DifferentiatorICPrevScaledInput=0  ExternalReset=none  TrackingMode=off  Kt=1  LimitOutput=off  UpperSaturationLimit=inf  LowerSaturationLimit=-inf  LinearizeAsGain=off  AntiWindupMode=none  Kb=1  POutMin=[]  POutMax=[]  IOutMin=[]  IOutMax=[]  DOutMin=[]  DOutMax=[]  NOutMin=[]  NOutMax=[]  SumOutMin=[]  SumOutMax=[]  SaturationOutMin=[]  SaturationOutMax=[]  PParamMin=[]  PParamMax=[]  IParamMin=[]  IParamMax=[]  DParamMin=[]  DParamMax=[]  NParamMin=[]  NParamMax=[]  KbParamMin=[]  KbParamMax=[]  KtParamMin=[]  KtParamMax=[]  KbOutMin=[]  KbOutMax=[]  KtOutMin=[]  KtOutMax=[]  IntegratorOutMin=[]  IntegratorOutMax=[]  FilterOutMin=[]  FilterOutMax=[]  SumI1OutMin=[]  SumI1OutMax=[]  SumI2OutMin=[]  SumI2OutMax=[]  SumI3OutMin=[]  SumI3OutMax=[]  SumI4OutMin=[]  SumI4OutMax=[]  SumDOutMin=[]  SumDOutMax=[]  DifferentiatorOutMin=[]  DifferentiatorOutMax=[]  FilterDiffOutCoefMin=[]  FilterDiffOutCoefMax=[]  ReciprocalOutMin=[]  ReciprocalOutMax=[]  SumDenOutMin=[]  SumDenOutMax=[]  SumNumOutMin=[]  SumNumOutMax=[]  DivideOutMin=[]  DivideOutMax=[]  UdiffTsProdOutMin=[]  UdiffTsProdOutMax=[]  NTsProdOutMin=[]  NTsProdOutMax=[]  UintegralTsProdOutMin=[]  UintegralTsProdOutMax=[]  UngainTsProdOutMin=[]  UngainTsProdOutMax=[]  IntegratorContinuousStateAttributes=''  IntegratorStateMustResolveToSignalObject=off  IntegratorRTWStateStorageClass=Auto  FilterContinuousStateAttributes=''  FilterStateMustResolveToSignalObject=off  FilterRTWStateStorageClass=Auto  ParallelPVariant=InternalParameters  IdealPVariant=Disabled  IVariant=InternalParameters  DVariant=Disabled  IntegratorVariant=Discrete  SatVariant=Disabled  AWVariant=Passthrough  PCopyVariant=Disabled  TRVariant=Disabled  FdbkBlocksVariant=Forward  IdealPFdbkVariant=Disabled  SatFdbkVariant=Disabled  DerivativeFilterVariant=Disabled  NVariant=Disabled  NCopyVariant=Disabled_SignalSpec  FilterICVariant=Disabled  IntegratorICVariant=InternalICs  ExternalResetVariant=Disabled  TRSumVariant=Passthrough  SumFdbkVariant=Disabled  SumVariant=Sum_PI  TsampFilterVariant=InternalTs  TsampNgainVariant=Passthrough  TsampIntegralVariant=Passthrough
  PI_8 : simulink/Continuous/PID Controller  Controller=PI  Form=Parallel  TimeDomain=Discrete-time  UseExternalTs=off  SampleTime=-1  IntegratorMethod=Forward Euler  FilterMethod=Forward Euler  ControllerParametersSource=internal  P=0.0417  I=-0.331  D=0  UseFilter=on  N=100  TunerSelectOption=Transfer Function Based (PID Tuner App)  InitialConditionSource=internal  InitialConditionForIntegrator=0  InitialConditionForFilter=0  DifferentiatorICPrevScaledInput=0  ExternalReset=none  TrackingMode=off  Kt=1  LimitOutput=off  UpperSaturationLimit=inf  LowerSaturationLimit=-inf  LinearizeAsGain=off  AntiWindupMode=none  Kb=1  POutMin=[]  POutMax=[]  IOutMin=[]  IOutMax=[]  DOutMin=[]  DOutMax=[]  NOutMin=[]  NOutMax=[]  SumOutMin=[]  SumOutMax=[]  SaturationOutMin=[]  SaturationOutMax=[]  PParamMin=[]  PParamMax=[]  IParamMin=[]  IParamMax=[]  DParamMin=[]  DParamMax=[]  NParamMin=[]  NParamMax=[]  KbParamMin=[]  KbParamMax=[]  KtParamMin=[]  KtParamMax=[]  KbOutMin=[]  KbOutMax=[]  KtOutMin=[]  KtOutMax=[]  IntegratorOutMin=[]  IntegratorOutMax=[]  FilterOutMin=[]  FilterOutMax=[]  SumI1OutMin=[]  SumI1OutMax=[]  SumI2OutMin=[]  SumI2OutMax=[]  SumI3OutMin=[]  SumI3OutMax=[]  SumI4OutMin=[]  SumI4OutMax=[]  SumDOutMin=[]  SumDOutMax=[]  DifferentiatorOutMin=[]  DifferentiatorOutMax=[]  FilterDiffOutCoefMin=[]  FilterDiffOutCoefMax=[]  ReciprocalOutMin=[]  ReciprocalOutMax=[]  SumDenOutMin=[]  SumDenOutMax=[]  SumNumOutMin=[]  SumNumOutMax=[]  DivideOutMin=[]  DivideOutMax=[]  UdiffTsProdOutMin=[]  UdiffTsProdOutMax=[]  NTsProdOutMin=[]  NTsProdOutMax=[]  UintegralTsProdOutMin=[]  UintegralTsProdOutMax=[]  UngainTsProdOutMin=[]  UngainTsProdOutMax=[]  IntegratorContinuousStateAttributes=''  IntegratorStateMustResolveToSignalObject=off  IntegratorRTWStateStorageClass=Auto  FilterContinuousStateAttributes=''  FilterStateMustResolveToSignalObject=off  FilterRTWStateStorageClass=Auto  ParallelPVariant=InternalParameters  IdealPVariant=Disabled  IVariant=InternalParameters  DVariant=Disabled  IntegratorVariant=Discrete  SatVariant=Disabled  AWVariant=Passthrough  PCopyVariant=Disabled  TRVariant=Disabled  FdbkBlocksVariant=Forward  IdealPFdbkVariant=Disabled  SatFdbkVariant=Disabled  DerivativeFilterVariant=Disabled  NVariant=Disabled  NCopyVariant=Disabled_SignalSpec  FilterICVariant=Disabled  IntegratorICVariant=InternalICs  ExternalResetVariant=Disabled  TRSumVariant=Passthrough  SumFdbkVariant=Disabled  SumVariant=Sum_PI  TsampFilterVariant=InternalTs  TsampNgainVariant=Passthrough  TsampIntegralVariant=Passthrough
  Pos : Step  Time=10  Before=30  After=60  SampleTime=0
  Scope : Scope  NumInputPorts=2
  Selector : Selector  InputPortWidth=6  IndexOptions=Index vector (dialog)  Indices=[2 4 6]  OutputSizes=1
  Selector1 : Selector  InputPortWidth=6  IndexOptions=Index vector (dialog)  Indices=[1 3 5]  OutputSizes=1
  Subsystem : Subsystem
  Sum : Sum  Inputs=|+-
  Vel : Step  Time=250  SampleTime=0
  dL : Step  Time=450  After=0.2  SampleTime=0
  dV : Step  Time=650  After=0.2  SampleTime=0
  wires:
  Selector/1 -> Scope/1  "D (tops)"
  Selector1/1 -> Scope/2  "B (bottoms)"
  Mux3/1 -> Selector/1, Selector1/1
  dL/1 -> Mux2/1
  OpenSim Plant/1(Out1) -> Mux3/3, Sum/2  "y"
  dV/1 -> Mux2/2
  Mux2/1 -> Mux3/2
  Mux/1 -> Sum/1, Mux3/1  "r"
  Sum/1 -> DM/1  "e"
  Pos/1 -> Degrees to Radians/1
  Vel/1 -> Degrees to Radians1/1
  Degrees to Radians/1 -> Mux/1
  Degrees to Radians1/1 -> Mux/2
  Demux1/7 -> PI_7/1
  PI_6/1 -> Mux4/6
  Demux1/4 -> PI_4/1
  Demux1/5 -> PI_5/1
  PI_8/1 -> Mux4/8
  PI_3/1 -> Mux4/3
  PI_7/1 -> Mux4/7
  Demux1/1 -> PI_1/1
  Demux1/2 -> PI_2/1
  PI_4/1 -> Mux4/4
  PI_2/1 -> Mux4/2
  PI_5/1 -> Mux4/5
  Demux1/6 -> PI_6/1
  Demux1/8 -> PI_8/1
  PI_1/1 -> Mux4/1
  Demux1/3 -> PI_3/1
  DM/1 -> Demux1/1
  Mux4/1 -> OpenSim Plant/1(In1)  "u"

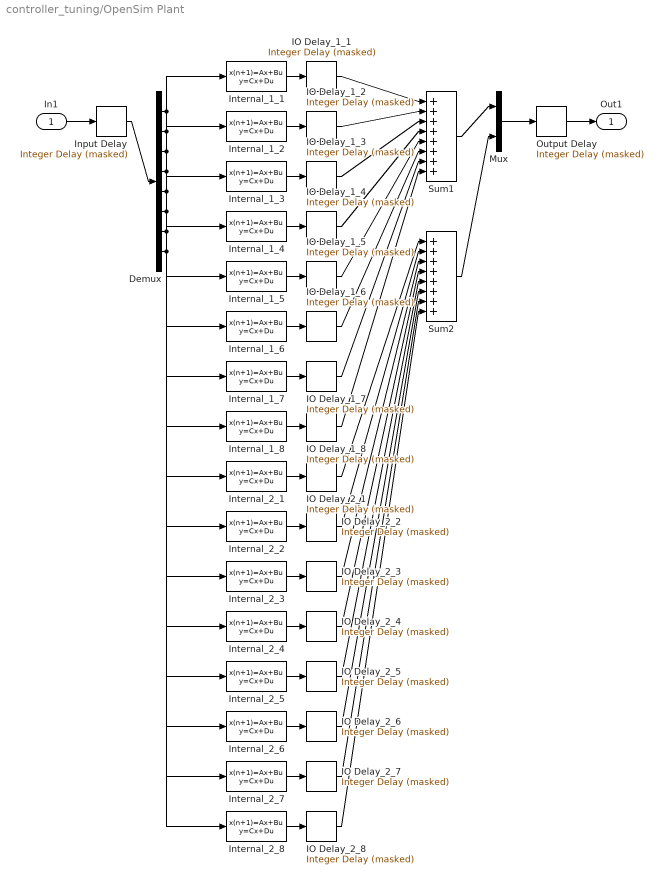
== system controller_tuning/OpenSim Plant ==
  In1 : Inport
  Demux : Demux  Outputs=8
  IO Delay_1_1 : cstextras/Integer Delay (masked)  Td=Tdio(1,1)  u0=0  Ts=Ts
      settings: SourceProductBaseCode=CT
  IO Delay_1_2 : cstextras/Integer Delay (masked)  Td=Tdio(1,2)  u0=0  Ts=Ts
      settings: SourceProductBaseCode=CT
  IO Delay_1_3 : cstextras/Integer Delay (masked)  Td=Tdio(1,3)  u0=0  Ts=Ts
      settings: SourceProductBaseCode=CT
  IO Delay_1_4 : cstextras/Integer Delay (masked)  Td=Tdio(1,4)  u0=0  Ts=Ts
      settings: SourceProductBaseCode=CT
  IO Delay_1_5 : cstextras/Integer Delay (masked)  Td=Tdio(1,5)  u0=0  Ts=Ts
      settings: SourceProductBaseCode=CT
  IO Delay_1_6 : cstextras/Integer Delay (masked)  Td=Tdio(1,6)  u0=0  Ts=Ts
      settings: SourceProductBaseCode=CT
  IO Delay_1_7 : cstextras/Integer Delay (masked)  Td=Tdio(1,7)  u0=0  Ts=Ts
      settings: SourceProductBaseCode=CT
  IO Delay_1_8 : cstextras/Integer Delay (masked)  Td=Tdio(1,8)  u0=0  Ts=Ts
      settings: SourceProductBaseCode=CT
  IO Delay_2_1 : cstextras/Integer Delay (masked)  Td=Tdio(2,1)  u0=0  Ts=Ts
      settings: SourceProductBaseCode=CT
  IO Delay_2_2 : cstextras/Integer Delay (masked)  Td=Tdio(2,2)  u0=0  Ts=Ts
      settings: SourceProductBaseCode=CT
  IO Delay_2_3 : cstextras/Integer Delay (masked)  Td=Tdio(2,3)  u0=0  Ts=Ts
      settings: SourceProductBaseCode=CT
  IO Delay_2_4 : cstextras/Integer Delay (masked)  Td=Tdio(2,4)  u0=0  Ts=Ts
      settings: SourceProductBaseCode=CT
  IO Delay_2_5 : cstextras/Integer Delay (masked)  Td=Tdio(2,5)  u0=0  Ts=Ts
      settings: SourceProductBaseCode=CT
  IO Delay_2_6 : cstextras/Integer Delay (masked)  Td=Tdio(2,6)  u0=0  Ts=Ts
      settings: SourceProductBaseCode=CT
  IO Delay_2_7 : cstextras/Integer Delay (masked)  Td=Tdio(2,7)  u0=0  Ts=Ts
      settings: SourceProductBaseCode=CT
  IO Delay_2_8 : cstextras/Integer Delay (masked)  Td=Tdio(2,8)  u0=0  Ts=Ts
      settings: SourceProductBaseCode=CT
  Input Delay : cstextras/Integer Delay (masked)  Td=Tdi  u0=0  Ts=Ts
      settings: SourceProductBaseCode=CT
  Internal_1_1 : DiscreteStateSpace  A=D(1,1).a  B=D(1,1).b  C=D(1,1).c  D=D(1,1).d  SampleTime=Ts
  Internal_1_2 : DiscreteStateSpace  A=D(1,2).a  B=D(1,2).b  C=D(1,2).c  D=D(1,2).d  SampleTime=Ts
  Internal_1_3 : DiscreteStateSpace  A=D(1,3).a  B=D(1,3).b  C=D(1,3).c  D=D(1,3).d  SampleTime=Ts
  Internal_1_4 : DiscreteStateSpace  A=D(1,4).a  B=D(1,4).b  C=D(1,4).c  D=D(1,4).d  SampleTime=Ts
  Internal_1_5 : DiscreteStateSpace  A=D(1,5).a  B=D(1,5).b  C=D(1,5).c  D=D(1,5).d  SampleTime=Ts
  Internal_1_6 : DiscreteStateSpace  A=D(1,6).a  B=D(1,6).b  C=D(1,6).c  D=D(1,6).d  SampleTime=Ts
  Internal_1_7 : DiscreteStateSpace  A=D(1,7).a  B=D(1,7).b  C=D(1,7).c  D=D(1,7).d  SampleTime=Ts
  Internal_1_8 : DiscreteStateSpace  A=D(1,8).a  B=D(1,8).b  C=D(1,8).c  D=D(1,8).d  SampleTime=Ts
  Internal_2_1 : DiscreteStateSpace  A=D(2,1).a  B=D(2,1).b  C=D(2,1).c  D=D(2,1).d  SampleTime=Ts
  Internal_2_2 : DiscreteStateSpace  A=D(2,2).a  B=D(2,2).b  C=D(2,2).c  D=D(2,2).d  SampleTime=Ts
  Internal_2_3 : DiscreteStateSpace  A=D(2,3).a  B=D(2,3).b  C=D(2,3).c  D=D(2,3).d  SampleTime=Ts
  Internal_2_4 : DiscreteStateSpace  A=D(2,4).a  B=D(2,4).b  C=D(2,4).c  D=D(2,4).d  SampleTime=Ts
  Internal_2_5 : DiscreteStateSpace  A=D(2,5).a  B=D(2,5).b  C=D(2,5).c  D=D(2,5).d  SampleTime=Ts
  Internal_2_6 : DiscreteStateSpace  A=D(2,6).a  B=D(2,6).b  C=D(2,6).c  D=D(2,6).d  SampleTime=Ts
  Internal_2_7 : DiscreteStateSpace  A=D(2,7).a  B=D(2,7).b  C=D(2,7).c  D=D(2,7).d  SampleTime=Ts
  Internal_2_8 : DiscreteStateSpace  A=D(2,8).a  B=D(2,8).b  C=D(2,8).c  D=D(2,8).d  SampleTime=Ts
  Mux : Mux  Inputs=2
  Output Delay : cstextras/Integer Delay (masked)  Td=Tdo  u0=0  Ts=Ts
      settings: SourceProductBaseCode=CT
  Sum1 : Sum  Inputs=++++++++
  Sum2 : Sum  Inputs=++++++++
  Out1 : Outport  InitialOutput=0  VectorParamsAs1DForOutWhenUnconnected=off
  wires:
  In1/1 -> Input Delay/1
  Output Delay/1 -> Out1/1
  Input Delay/1 -> Demux/1
  Mux/1 -> Output Delay/1
  Sum1/1 -> Mux/1
  Sum2/1 -> Mux/2
  Demux/1 -> Internal_1_1/1, Internal_2_1/1
  Internal_1_1/1 -> IO Delay_1_1/1
  IO Delay_1_1/1 -> Sum1/1
  Demux/2 -> Internal_1_2/1, Internal_2_2/1
  Internal_1_2/1 -> IO Delay_1_2/1
  IO Delay_1_2/1 -> Sum1/2
  Demux/3 -> Internal_1_3/1, Internal_2_3/1
  Internal_1_3/1 -> IO Delay_1_3/1
  IO Delay_1_3/1 -> Sum1/3
  Demux/4 -> Internal_1_4/1, Internal_2_4/1
  Internal_1_4/1 -> IO Delay_1_4/1
  IO Delay_1_4/1 -> Sum1/4
  Demux/5 -> Internal_1_5/1, Internal_2_5/1
  Internal_1_5/1 -> IO Delay_1_5/1
  IO Delay_1_5/1 -> Sum1/5
  Demux/6 -> Internal_1_6/1, Internal_2_6/1
  Internal_1_6/1 -> IO Delay_1_6/1
  IO Delay_1_6/1 -> Sum1/6
  Demux/7 -> Internal_1_7/1, Internal_2_7/1
  Internal_1_7/1 -> IO Delay_1_7/1
  IO Delay_1_7/1 -> Sum1/7
  Demux/8 -> Internal_1_8/1, Internal_2_8/1
  Internal_1_8/1 -> IO Delay_1_8/1
  IO Delay_1_8/1 -> Sum1/8
  Internal_2_1/1 -> IO Delay_2_1/1
  IO Delay_2_1/1 -> Sum2/1
  Internal_2_2/1 -> IO Delay_2_2/1
  IO Delay_2_2/1 -> Sum2/2
  Internal_2_3/1 -> IO Delay_2_3/1
  IO Delay_2_3/1 -> Sum2/3
  Internal_2_4/1 -> IO Delay_2_4/1
  IO Delay_2_4/1 -> Sum2/4
  Internal_2_5/1 -> IO Delay_2_5/1
  IO Delay_2_5/1 -> Sum2/5
  Internal_2_6/1 -> IO Delay_2_6/1
  IO Delay_2_6/1 -> Sum2/6
  Internal_2_7/1 -> IO Delay_2_7/1
  IO Delay_2_7/1 -> Sum2/7
  Internal_2_8/1 -> IO Delay_2_8/1
  IO Delay_2_8/1 -> Sum2/8

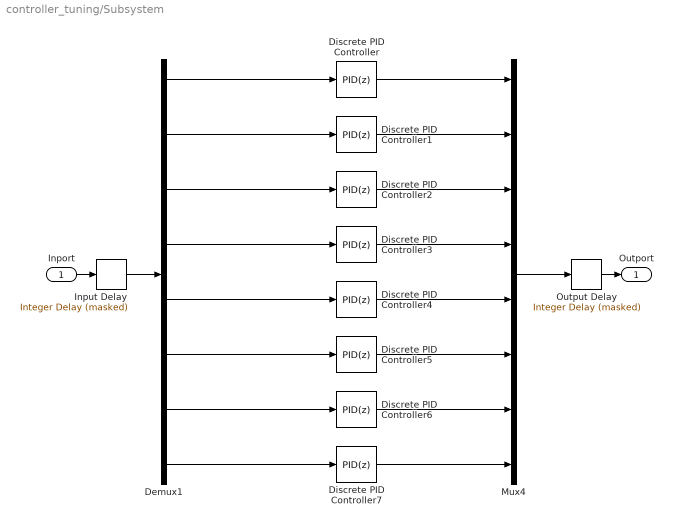
== system controller_tuning/Subsystem ==
  Inport : Inport
  Demux1 : Demux  Outputs=8
  Discrete PID Controller{,1..7} (8 alike) : simulink/Continuous/PID Controller  Controller=PID  Form=Parallel  TimeDomain=Discrete-time  UseExternalTs=off  SampleTime=-1  IntegratorMethod=Forward Euler  FilterMethod=Forward Euler  ControllerParametersSource=internal  P=1  I=1  D=0  UseFilter=on  N=100  TunerSelectOption=Transfer Function Based (PID Tuner App)  InitialConditionSource=internal  InitialConditionForIntegrator=0  InitialConditionForFilter=0  DifferentiatorICPrevScaledInput=0  ExternalReset=none  TrackingMode=off  Kt=1  LimitOutput=off  UpperSaturationLimit=inf  LowerSaturationLimit=-inf  LinearizeAsGain=off  AntiWindupMode=none  Kb=1  POutMin=[]  POutMax=[]  IOutMin=[]  IOutMax=[]  DOutMin=[]  DOutMax=[]  NOutMin=[]  NOutMax=[]  SumOutMin=[]  SumOutMax=[]  SaturationOutMin=[]  SaturationOutMax=[]  PParamMin=[]  PParamMax=[]  IParamMin=[]  IParamMax=[]  DParamMin=[]  DParamMax=[]  NParamMin=[]  NParamMax=[]  KbParamMin=[]  KbParamMax=[]  KtParamMin=[]  KtParamMax=[]  KbOutMin=[]  KbOutMax=[]  KtOutMin=[]  KtOutMax=[]  IntegratorOutMin=[]  IntegratorOutMax=[]  FilterOutMin=[]  FilterOutMax=[]  SumI1OutMin=[]  SumI1OutMax=[]  SumI2OutMin=[]  SumI2OutMax=[]  SumI3OutMin=[]  SumI3OutMax=[]  SumI4OutMin=[]  SumI4OutMax=[]  SumDOutMin=[]  SumDOutMax=[]  DifferentiatorOutMin=[]  DifferentiatorOutMax=[]  FilterDiffOutCoefMin=[]  FilterDiffOutCoefMax=[]  ReciprocalOutMin=[]  ReciprocalOutMax=[]  SumDenOutMin=[]  SumDenOutMax=[]  SumNumOutMin=[]  SumNumOutMax=[]  DivideOutMin=[]  DivideOutMax=[]  UdiffTsProdOutMin=[]  UdiffTsProdOutMax=[]  NTsProdOutMin=[]  NTsProdOutMax=[]  UintegralTsProdOutMin=[]  UintegralTsProdOutMax=[]  UngainTsProdOutMin=[]  UngainTsProdOutMax=[]  IntegratorContinuousStateAttributes=''  IntegratorStateMustResolveToSignalObject=off  IntegratorRTWStateStorageClass=Auto  FilterContinuousStateAttributes=''  FilterStateMustResolveToSignalObject=off  FilterRTWStateStorageClass=Auto  ParallelPVariant=InternalParameters  IdealPVariant=Disabled  IVariant=InternalParameters  DVariant=InternalParameters  IntegratorVariant=Discrete  SatVariant=Disabled  AWVariant=Passthrough  PCopyVariant=Disabled  TRVariant=Disabled  FdbkBlocksVariant=Forward  IdealPFdbkVariant=Disabled  SatFdbkVariant=Disabled  DerivativeFilterVariant=ForwardEulerFilter  NVariant=InternalParameters  NCopyVariant=Disabled  FilterICVariant=InternalICsFilter  IntegratorICVariant=InternalICs  ExternalResetVariant=Disabled  TRSumVariant=Passthrough  SumFdbkVariant=Disabled  SumVariant=Sum_PID  TsampFilterVariant=InternalTs  TsampNgainVariant=Passthrough  TsampIntegralVariant=Passthrough
  Input Delay : cstextras/Integer Delay (masked)  Td=Tdi  u0=0  Ts=Ts
      settings: SourceProductBaseCode=CT
  Mux4 : Mux  Inputs=8
  Output Delay : cstextras/Integer Delay (masked)  Td=Tdo  u0=0  Ts=Ts
      settings: SourceProductBaseCode=CT
  Outport : Outport
  wires:
  Discrete PID Controller/1 -> Mux4/1
  Mux4/1 -> Output Delay/1
  Discrete PID Controller5/1 -> Mux4/6
  Discrete PID Controller3/1 -> Mux4/4
  Demux1/4 -> Discrete PID Controller3/1
  Input Delay/1 -> Demux1/1
  Discrete PID Controller1/1 -> Mux4/2
  Demux1/1 -> Discrete PID Controller/1
  Demux1/6 -> Discrete PID Controller5/1
  Discrete PID Controller4/1 -> Mux4/5
  Demux1/2 -> Discrete PID Controller1/1
  Discrete PID Controller7/1 -> Mux4/8
  Demux1/7 -> Discrete PID Controller6/1
  Demux1/8 -> Discrete PID Controller7/1
  Discrete PID Controller6/1 -> Mux4/7
  Output Delay/1 -> Outport/1
  Demux1/5 -> Discrete PID Controller4/1
  Discrete PID Controller2/1 -> Mux4/3
  Demux1/3 -> Discrete PID Controller2/1
  Inport/1 -> Input Delay/1
